simulink model "DC_motor_resonant_load"  (R2024b)
settings: Solver=VariableStepAuto  StartTime=0.0  StopTime=10.0  RelTol=1e-3
values from neighbouring files (symbols this model uses):
  Beq = mot.B+(mld.Bh)/((gbox.N)^2)    [LQR_code.m]
  Jb = 1.4e-3    (= 0.0014)    [Elastic_parameters_estimation.m]
  N = linsolve(SYS,f)    [LQR_code.m]
  Req = sens.curr.Rs+mot.R    [LQR_code.m]
undefined symbols (not defined in the file or in its folder): Bb, daq, deg2V, drv, Jeq_hat, k, k_drv, Ke, Kt, mot, rads2rpm, sens, T_drv, tau_sf, V2deg
settings Model: Creator=lucag  LastModifiedBy=lucag

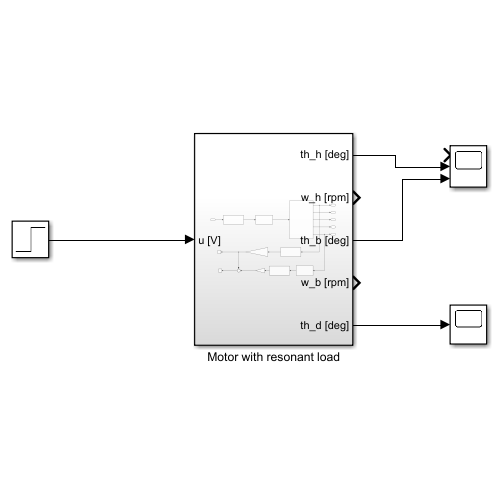
[thumbnail: Simulink's stored preview of the top-level diagram]
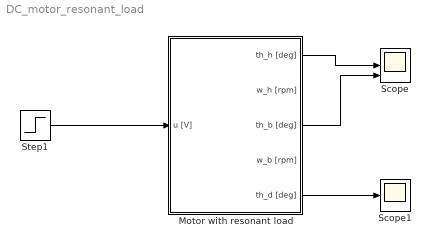
== system DC_motor_resonant_load ==
  Motor with resonant load : Subsystem
  Scope : Scope  NumInputPorts=3
  Scope1 : Scope
  Step1 : Step  Time=1.1  After=5  SampleTime=0
  wires:
  Motor with resonant load/1(th_h [deg]) -> Scope/2
  Motor with resonant load/3(th_b [deg]) -> Scope/3
  Motor with resonant load/5(th_d [deg]) -> Scope1/1
  Step1/1 -> Motor with resonant load/1(u [V])

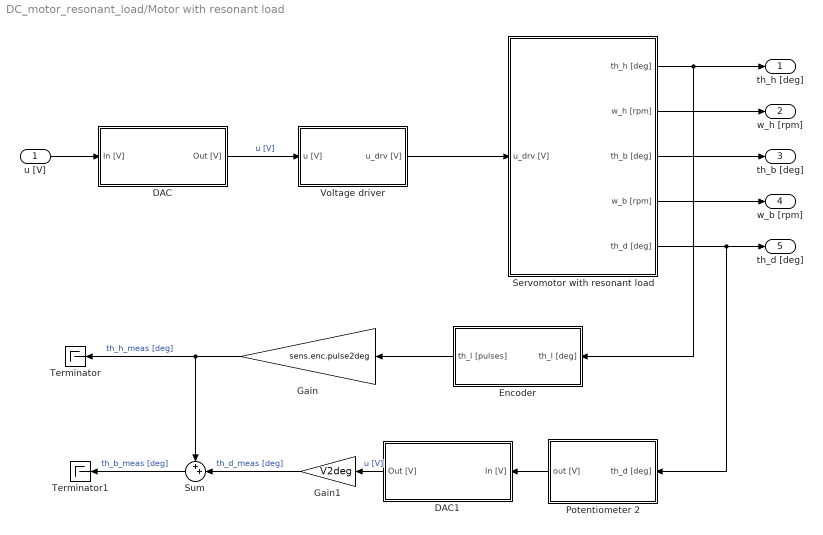
== system DC_motor_resonant_load/Motor with resonant load ==
  u [V] : Inport
  DAC : Subsystem
  DAC1 : Subsystem
  Encoder : Subsystem
  Gain : Gain  Gain=sens.enc.pulse2deg
  Gain1 : Gain  Gain=V2deg
  Potentiometer 2 : Subsystem
  Servomotor with resonant load : Subsystem
  Sum : Sum  Inputs=++|
  Terminator : Terminator
  Terminator1 : Terminator
  Voltage driver : Subsystem
  th_h [deg] : Outport
  w_h [rpm] : Outport  Port=2
  th_b [deg] : Outport  Port=3
  w_b [rpm] : Outport  Port=4
  th_d [deg] : Outport  Port=5
  wires:
  Encoder/1(th_l [pulses]) -> Gain/1
  u [V]/1 -> DAC/1(In [V])
  DAC/1(Out [V]) -> Voltage driver/1(u [V])  "u [V]"
  Voltage driver/1(u_drv [V]) -> Servomotor with resonant load/1(u_drv [V])
  Servomotor with resonant load/1(th_h [deg]) -> Encoder/1(th_l [deg]), th_h [deg]/1
  Servomotor with resonant load/2(w_h [rpm]) -> w_h [rpm]/1
  Servomotor with resonant load/3(th_b [deg]) -> th_b [deg]/1
  Servomotor with resonant load/4(w_b [rpm]) -> w_b [rpm]/1
  Servomotor with resonant load/5(th_d [deg]) -> Potentiometer 2/1(th_d [deg]), th_d [deg]/1
  Gain/1 -> Terminator/1, Sum/1  "th_h_meas [deg]"
  Potentiometer 2/1(out [V]) -> DAC1/1(In [V])
  DAC1/1(Out [V]) -> Gain1/1  "u [V]"
  Gain1/1 -> Sum/2  "th_d_meas [deg]"
  Sum/1 -> Terminator1/1  "th_b_meas [deg]"

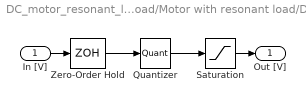
== system DC_motor_resonant_load/Motor with resonant load/DAC ==
  In [V] : Inport
  Quantizer : Quantizer  QuantizationInterval=daq.dac.q
  Saturation : Saturate  UpperLimit=daq.dac.fs  LowerLimit=-daq.dac.fs
  Zero-Order Hold : ZeroOrderHold  SampleTime=1e-3
  Out [V] : Outport
  wires:
  Saturation/1 -> Out [V]/1
  Zero-Order Hold/1 -> Quantizer/1
  Quantizer/1 -> Saturation/1
  In [V]/1 -> Zero-Order Hold/1

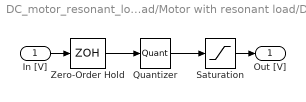
== system DC_motor_resonant_load/Motor with resonant load/DAC1 ==
  In [V] : Inport
  Quantizer : Quantizer  QuantizationInterval=daq.dac.q
  Saturation : Saturate  UpperLimit=daq.dac.fs  LowerLimit=-daq.dac.fs
  Zero-Order Hold : ZeroOrderHold  SampleTime=1e-3
  Out [V] : Outport
  wires:
  In [V]/1 -> Zero-Order Hold/1
  Quantizer/1 -> Saturation/1
  Zero-Order Hold/1 -> Quantizer/1
  Saturation/1 -> Out [V]/1

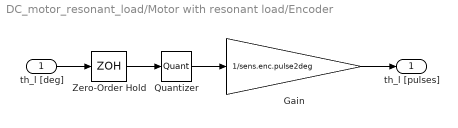
== system DC_motor_resonant_load/Motor with resonant load/Encoder ==
  th_l [deg] : Inport
  Gain : Gain  Gain=1/sens.enc.pulse2deg
  Quantizer : Quantizer  QuantizationInterval=sens.enc.pulse2deg
  Zero-Order Hold : ZeroOrderHold  SampleTime=1e-3
  th_l [pulses] : Outport
  wires:
  th_l [deg]/1 -> Zero-Order Hold/1
  Quantizer/1 -> Gain/1
  Zero-Order Hold/1 -> Quantizer/1
  Gain/1 -> th_l [pulses]/1

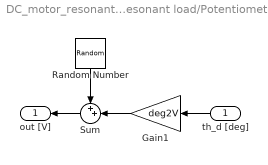
== system DC_motor_resonant_load/Motor with resonant load/Potentiometer 2 ==
  th_d [deg] : Inport
  Gain1 : Gain  Gain=deg2V
  Random Number : RandomNumber  Variance=sens.pot2.noise.var  SampleTime=1e-3
  Sum : Sum  Inputs=++|
  out [V] : Outport
  wires:
  Gain1/1 -> Sum/2
  th_d [deg]/1 -> Gain1/1
  Random Number/1 -> Sum/1
  Sum/1 -> out [V]/1

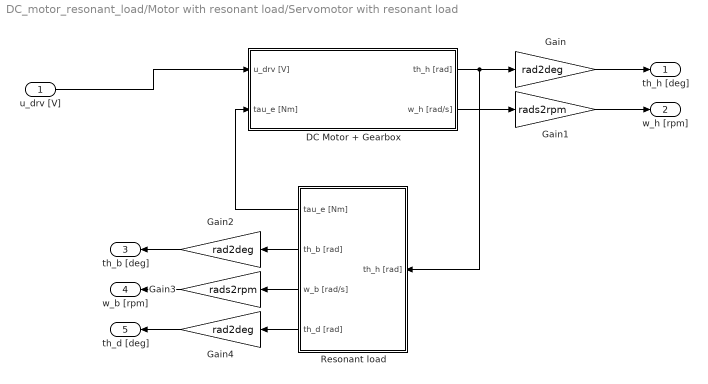
== system DC_motor_resonant_load/Motor with resonant load/Servomotor with resonant load ==
  u_drv [V] : Inport
  DC Motor + Gearbox : Subsystem
  Gain : Gain  Gain=rad2deg
  Gain1 : Gain  Gain=rads2rpm
  Gain2 : Gain  Gain=rad2deg
  Gain3 : Gain  Gain=rads2rpm
  Gain4 : Gain  Gain=rad2deg
  Resonant load : Subsystem
  th_h [deg] : Outport
  w_h [rpm] : Outport  Port=2
  th_b [deg] : Outport  Port=3
  w_b [rpm] : Outport  Port=4
  th_d [deg] : Outport  Port=5
  wires:
  Resonant load/1(tau_e [Nm]) -> DC Motor + Gearbox/2(tau_e [Nm])
  Gain4/1 -> th_d [deg]/1
  Gain2/1 -> th_b [deg]/1
  Resonant load/2(th_b [rad]) -> Gain2/1
  DC Motor + Gearbox/2(w_h [rad/s]) -> Gain1/1
  DC Motor + Gearbox/1(th_h [rad]) -> Gain/1, Resonant load/1(th_h [rad])
  Resonant load/3(w_b [rad/s]) -> Gain3/1
  Gain1/1 -> w_h [rpm]/1
  Resonant load/4(th_d [rad]) -> Gain4/1
  Gain/1 -> th_h [deg]/1
  Gain3/1 -> w_b [rpm]/1
  u_drv [V]/1 -> DC Motor + Gearbox/1(u_drv [V])

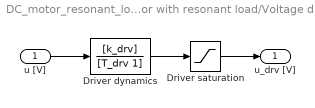
== system DC_motor_resonant_load/Motor with resonant load/Voltage driver ==
  u [V] : Inport
  Driver dynamics : TransferFcn  Numerator=[k_drv]  Denominator=[T_drv 1]
  Driver saturation : Saturate  UpperLimit=drv.outmax  LowerLimit=-drv.outmax
  u_drv [V] : Outport
  wires:
  Driver dynamics/1 -> Driver saturation/1
  Driver saturation/1 -> u_drv [V]/1
  u [V]/1 -> Driver dynamics/1

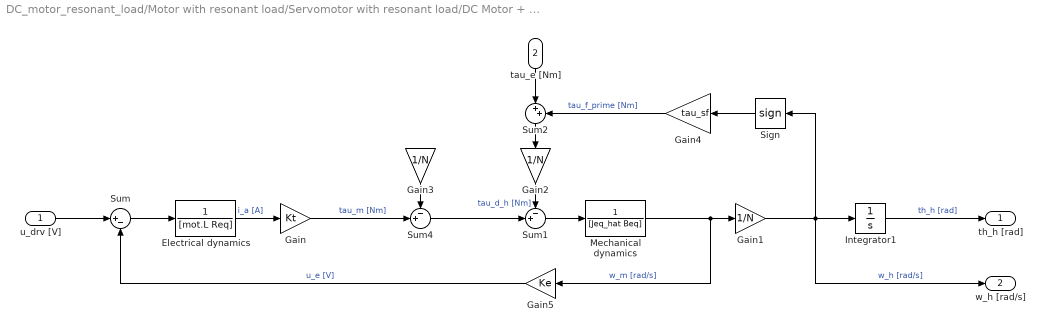
== system DC_motor_resonant_load/Motor with resonant load/Servomotor with resonant load/DC Motor + Gearbox ==
  u_drv [V] : Inport
  tau_e [Nm] : Inport  Port=2
  Electrical dynamics : TransferFcn  Denominator=[mot.L Req]
  Gain : Gain  Gain=Kt
  Gain1 : Gain  Gain=1/N
  Gain2 : Gain  Gain=1/N
  Gain3 : Gain  Gain=1/N
  Gain4 : Gain  Gain=tau_sf
  Gain5 : Gain  Gain=Ke
  Integrator1 : Integrator
  Mechanical dynamics : TransferFcn  Denominator=[Jeq_hat Beq]
  Sign : Signum  ZeroCross=off
  Sum : Sum  Inputs=|+-
  Sum1 : Sum  Inputs=-+|
  Sum2 : Sum  Inputs=|++
  Sum4 : Sum  Inputs=-+|
  th_h [rad] : Outport
  w_h [rad/s] : Outport  Port=2
  wires:
  Integrator1/1 -> th_h [rad]/1  "th_h [rad]"
  Gain5/1 -> Sum/2  "u_e [V]"
  Gain1/1 -> Sign/1, w_h [rad/s]/1, Integrator1/1  "w_h [rad/s]"
  Electrical dynamics/1 -> Gain/1  "i_a [A]"
  Sign/1 -> Gain4/1
  Sum/1 -> Electrical dynamics/1
  Sum1/1 -> Mechanical dynamics/1
  Gain/1 -> Sum4/2  "tau_m [Nm]"
  Mechanical dynamics/1 -> Gain5/1, Gain1/1  "w_m [rad/s]"
  u_drv [V]/1 -> Sum/1
  Gain4/1 -> Sum2/2  "tau_f_prime [Nm]"
  Sum2/1 -> Gain2/1
  tau_e [Nm]/1 -> Sum2/1
  Gain2/1 -> Sum1/1  "tau_d_h [Nm]"
  Sum4/1 -> Sum1/2
  Gain3/1 -> Sum4/1

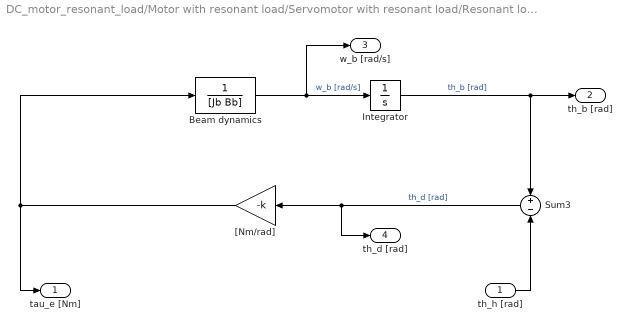
== system DC_motor_resonant_load/Motor with resonant load/Servomotor with resonant load/Resonant load ==
  th_h [rad] : Inport
  Beam dynamics : TransferFcn  Denominator=[Jb Bb]
  Integrator : Integrator
  Sum3 : Sum  Inputs=+|-
  "[Nm/rad]" : Gain  Gain=-k
  tau_e [Nm] : Outport
  th_b [rad] : Outport  Port=2
  w_b [rad/s] : Outport  Port=3
  th_d [rad] : Outport  Port=4
  wires:
  Integrator/1 -> th_b [rad]/1, Sum3/1  "th_b [rad]"
  "[Nm/rad]"/1 -> tau_e [Nm]/1, Beam dynamics/1
  Sum3/1 -> th_d [rad]/1, "[Nm/rad]"/1  "th_d [rad]"
  Beam dynamics/1 -> w_b [rad/s]/1, Integrator/1  "w_b [rad/s]"
  th_h [rad]/1 -> Sum3/2
